simulink model "MovimientoRotT"  (R2023b)
settings: Solver=ode23s  StartTime=0.0  StopTime=15  RelTol=1e-3
values from neighbouring files (symbols this model uses):
  k = 100    [MRT.mat]    (also in MovimientoRotTra.m)
  m = 10    [MRT.mat]    (also in MovimientoRotTra.m)
  r = 0.05    [MRT.mat]    (also in MovimientoRotTra.m)

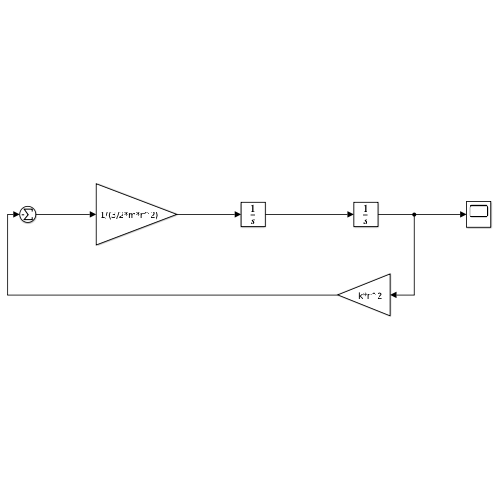
[thumbnail: Simulink's stored preview of the top-level diagram]
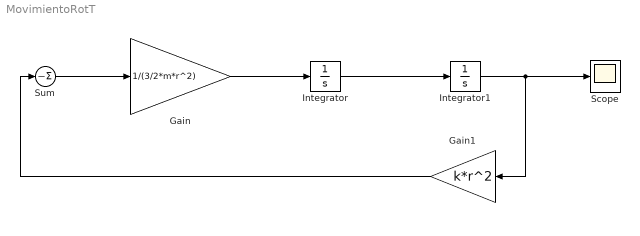
== system MovimientoRotT ==
  Gain : Gain  Gain=1/(3/2*m*r^2)
  Gain1 : Gain  Gain=k*r^2
  Integrator : Integrator  InitialCondition=2
  Integrator1 : Integrator
  Scope : Scope
  Sum : Sum  Inputs=-
  wires:
  Integrator/1 -> Integrator1/1
  Integrator1/1 -> Gain1/1, Scope/1
  Sum/1 -> Gain/1
  Gain/1 -> Integrator/1
  Gain1/1 -> Sum/1
